simulink model "soc_rfsoc_proc"  (R2025b)
settings: Solver=FixedStepAuto  StartTime=0.0  StopTime=10.0  RelTol=1e-3  EnableMultiTasking=on
model workspace (MAT data in the model file):
  SrcSel = 0
undefined symbols (not defined in the file): FrameSize
libraries: simulink x4, prociolib x2
settings Model: Creator=The MathWorks, Inc.  LastModifiedBy=The MathWorks, Inc.
settings SolverCC: AlgebraicLoopSolver=TrustRegion  PositivePriorityOrder=on
settings DataIOCC: SaveFormat=StructureWithTime  ReturnWorkspaceOutputs=off
settings OptimizationCC: PassReuseOutputArgsAs=Individual arguments  ZeroExternalMemoryAtStartup=off  MaxStackSize=64  EfficientTunableParamExpr=on
settings DebuggingCC: IntegerOverflowMsg=none  ParameterTunabilityLossMsg=error  UnconnectedInputMsg=warning  UnconnectedOutputMsg=warning  UnconnectedLineMsg=warning  ArithmeticOperatorsInVariantConditions=warning
settings HardwareCC: ProdBitPerLong=64.0  ProdLargestAtomicInteger=LongLong  ProdLargestAtomicFloat=Double  ProdLongLongMode=on  ProdHWDeviceType=ARM Compatible->ARM Cortex-A (64-bit)  HardwareBoardFeatureSet=SoCBlockset
settings ModelReferenceCC: EnableRefExpFcnMdlSchedulingChecks=on  ModelReferenceNumInstancesAllowed=Single
settings SFSimCC: SimUseLocalCustomCode=off
settings RTWCC: SystemTargetFile=ert.tlc  HardwareBoard=Xilinx Zynq UltraScale+ RFSoC ZCU111 Evaluation Kit  TLCOptions="-aInlineSetEventsForThisBaseRateFcn=TLC_FALSE -aSuppressMultiTaskScheduler=TLC_FALSE  -aRateBasedStepFcn=0"  GenCodeOnly=on  TemplateMakefile=ert_default_tmf  GenerateReport=on  RTWUseLocalCustomCode=off  Toolchain=Linaro AArch64 Linux v6.3.1  IncludeHyperlinkInReport=on  LaunchReport=on  GenerateTraceInfo=on  GenerateTraceReport=on  GenerateTraceReportSl=on  GenerateTraceReportSf=on  GenerateTraceReportEml=on  GPUComputeCapability=3.5  DLArmComputeVersion=19.05  Description=Embedded Coder
settings CodeAppCC: ForceParamTrailComments=on  IgnoreCustomStorageClasses=off  OperatorAnnotations=on  SimulinkDataObjDesc=on  SFDataObjDesc=on  InsertBlockDesc=on
settings ERTTargetCC: InlinedParameterPlacement=Hierarchical  DynamicArrayContainerType=coder::array  SubcomponentCodeInterfacePackaging=Nonreusable function

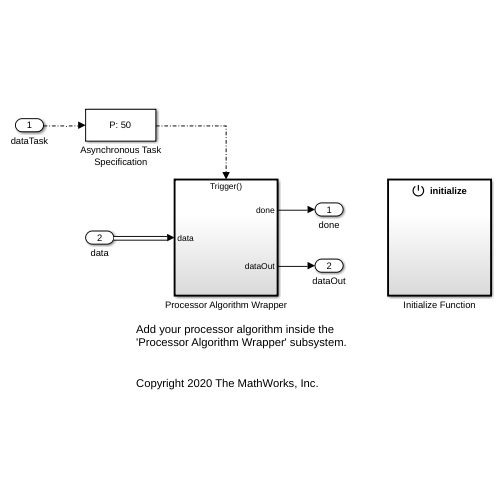
[thumbnail: Simulink's stored preview of the top-level diagram]
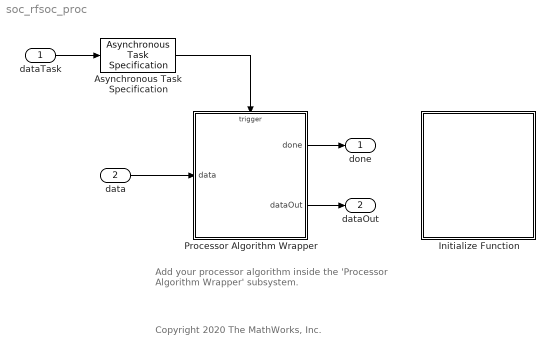
== system soc_rfsoc_proc ==
  note: Add your processor algorithm inside the
      | 'Processor Algorithm Wrapper' subsystem.
  note: Copyright 2020 The MathWorks, Inc.
  dataTask : Inport  OutputFunctionCall=on
  data : Inport  OutputPortMessageModes=m  Port=2  OutDataTypeStr=SoCData  BusOutputAsStruct=on
  Asynchronous Task Specification : AsynchronousTaskSpecification  TaskPriority=50
  Initialize Function : Subsystem  TreatAsAtomicUnit=on
  Processor Algorithm Wrapper : Subsystem  TreatAsAtomicUnit=on
  done : Outport  VectorParamsAs1DForOutWhenUnconnected=off  BusOutputAsStruct=on
  dataOut : Outport  Port=2  VectorParamsAs1DForOutWhenUnconnected=off
  wires:
  dataTask/1 -> Asynchronous Task Specification/1
  data/1 -> Processor Algorithm Wrapper/1(data)
  Processor Algorithm Wrapper/1(done) -> done/1
  Processor Algorithm Wrapper/2(dataOut) -> dataOut/1
  Asynchronous Task Specification/1 -> Processor Algorithm Wrapper/Trigger

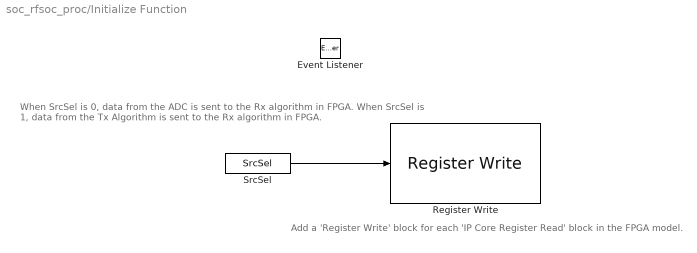
== system soc_rfsoc_proc/Initialize Function ==
  note: Add a 'Register Write' block for each 'IP Core Register Read' block in the FPGA model.
  note: When SrcSel is 0, data from the ADC is sent to the Rx algorithm in FPGA.
      | When SrcSel is 1, data from the Tx Algorithm is sent to the Rx algorithm in FPGA.
  Event Listener : EventListener  DisableCoverage=on  EventName=reset
  Register Write : prociolib/Register Write  OutputSink=IP core register  TunableParamName=A  RegisterName=SrcSelReg  DeviceName=/dev/mwipcore  OffsetAddress=hex2dec('100')  Dummy=0
  SrcSel : Constant  Value=SrcSel  OutDataTypeStr=boolean  SampleTime=-1
  wires:
  SrcSel/1 -> Register Write/1

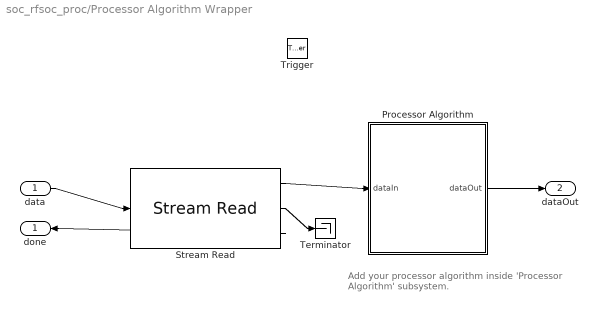
== system soc_rfsoc_proc/Processor Algorithm Wrapper ==
  note: Add your processor algorithm inside
      | 'Processor Algorithm' subsystem.
  data : Inport
  Trigger : TriggerPort  TriggerType=function-call  VariantControl=Variant  PortDimensions=1
  Processor Algorithm : Subsystem
  Stream Read : prociolib/Stream Read  DeviceName=ip:s2mm  OutDataTypeStr=uint64  SamplesPerFrame=FrameSize  NumberOfBuffers=NumBuffers  EnableEvent=on  SampleTime=-1
  Terminator : Terminator
  done : Outport  VectorParamsAs1DForOutWhenUnconnected=off
  dataOut : Outport  Port=2  VectorParamsAs1DForOutWhenUnconnected=off
  wires:
  data/1 -> Stream Read/1
  Stream Read/3 -> done/1
  Processor Algorithm/1(dataOut) -> dataOut/1
  Stream Read/1 -> Processor Algorithm/1(dataIn)
  Stream Read/2 -> Terminator/1

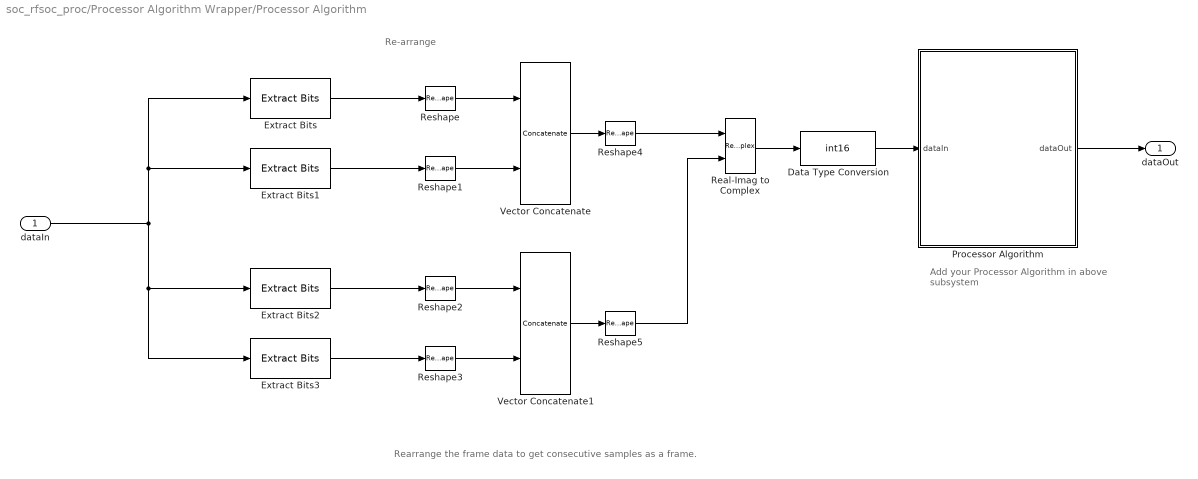
== system soc_rfsoc_proc/Processor Algorithm Wrapper/Processor Algorithm ==
  note: Rearrange the frame data to get consecutive samples as a frame.
  note: Re-arrange
  note: Add your Processor Algorithm in above subsystem
  dataIn : Inport
  Data Type Conversion : DataTypeConversion  OutDataTypeStr=int16  SaturateOnIntegerOverflow=off  RndMeth=Floor
  Extract Bits : simulink/Logic and Bit Operations/Extract Bits  bitsToExtract=Range of bits  numBits=8  bitIdxRange=[0 15]  outScalingMode=Treat bit field as an integer
  Extract Bits1 : simulink/Logic and Bit Operations/Extract Bits  bitsToExtract=Range of bits  numBits=8  bitIdxRange=[16 31]  outScalingMode=Treat bit field as an integer
  Extract Bits2 : simulink/Logic and Bit Operations/Extract Bits  bitsToExtract=Range of bits  numBits=8  bitIdxRange=[32 47]  outScalingMode=Treat bit field as an integer
  Extract Bits3 : simulink/Logic and Bit Operations/Extract Bits  bitsToExtract=Range of bits  numBits=8  bitIdxRange=[48 63]  outScalingMode=Treat bit field as an integer
  Processor Algorithm : Subsystem
  Real-Imag to Complex : RealImagToComplex
  Reshape{,1..3} (4 alike) : Reshape  OutputDimensionality=Customize  OutputDimensions=[1,FrameSize]
  Reshape4 : Reshape  OutputDimensionality=Customize  OutputDimensions=[2*FrameSize,1]
  Reshape5 : Reshape  OutputDimensionality=Customize  OutputDimensions=[2*FrameSize,1]
  Vector Concatenate : Concatenate  Mode=Multidimensional array
  Vector Concatenate1 : Concatenate  Mode=Multidimensional array
  dataOut : Outport  VectorParamsAs1DForOutWhenUnconnected=off
  wires:
  Real-Imag to Complex/1 -> Data Type Conversion/1
  Processor Algorithm/1(dataOut) -> dataOut/1
  Reshape4/1 -> Real-Imag to Complex/1
  Vector Concatenate/1 -> Reshape4/1
  Reshape/1 -> Vector Concatenate/1
  Reshape1/1 -> Vector Concatenate/2
  Reshape3/1 -> Vector Concatenate1/2
  Vector Concatenate1/1 -> Reshape5/1
  Reshape2/1 -> Vector Concatenate1/1
  Reshape5/1 -> Real-Imag to Complex/2
  dataIn/1 -> Extract Bits2/1, Extract Bits3/1, Extract Bits/1, Extract Bits1/1
  Data Type Conversion/1 -> Processor Algorithm/1(dataIn)
  Extract Bits/1 -> Reshape/1
  Extract Bits1/1 -> Reshape1/1
  Extract Bits2/1 -> Reshape2/1
  Extract Bits3/1 -> Reshape3/1

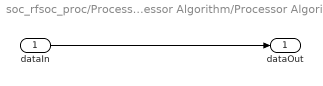
== system soc_rfsoc_proc/Processor Algorithm Wrapper/Processor Algorithm/Processor Algorithm ==
  dataIn : Inport
  dataOut : Outport  VectorParamsAs1DForOutWhenUnconnected=off
  wires:
  dataIn/1 -> dataOut/1
